simulink model "kopter_se_zavazim_state_feedback"  (R2024b)
settings: Solver=FixedStepAuto  StartTime=0.0  StopTime=30  FixedStep=0.01  RelTol=1e-3
values from neighbouring files (symbols this model uses):
  b_moment = 5.4e-6    (= 5.4e-06)    [parametry_kopter_se_zavazim.m]
  d = 1    [parametry_kopter_se_zavazim.m]
  g = 9.81    [parametry_kopter_se_zavazim.m]
  Ip = m*d^2    (= 1)    [parametry_kopter_se_zavazim.m]
  Ixx = 0.0222    [parametry_kopter_se_zavazim.m]
  Iyy = 0.0222    [parametry_kopter_se_zavazim.m]
  Izz = 0.0429    [parametry_kopter_se_zavazim.m]
  k_thrust = 2.3e-3    (= 0.0023)    [parametry_kopter_se_zavazim.m]
  ki = K_ex(:,17:20)    [odvozeni_stavova_regulace.m]
  ki_oa = K_ex_other_angles(:,17:20)    [odvozeni_stavova_regulace_OTHER_ANGLES.m]
  kp = K_ex(:, 1:16)    [odvozeni_stavova_regulace.m]
  kp_oa = K_ex_other_angles(:, 1:16)    [odvozeni_stavova_regulace_OTHER_ANGLES.m]
  M = 2    [parametry_kopter_se_zavazim.m]
  m = 1    [parametry_kopter_se_zavazim.m]
  Us_p = [(M+m)*g; 0; 0; 0]    [parametry_kopter_se_zavazim.m]
  Xinit_ss = [Xinit_matrix; [0 0 0 0 0 0 0 0]']    [parametry_kopter_se_zavazim.m]
  Xs_p = [0;0;0; 0;0;0; 0;0; 0;0;0; 0;0;0; 0;0]    [parametry_kopter_se_zavazim.m]
undefined symbols (not defined in the file or in its folder): L
libraries: simulink_extras x10
(part 1 of 6)
settings Model: Creator=Admin  LastModifiedBy=Admin

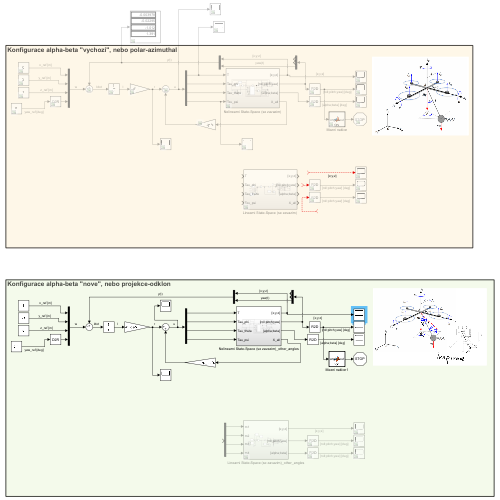
[thumbnail: Simulink's stored preview of the top-level diagram]
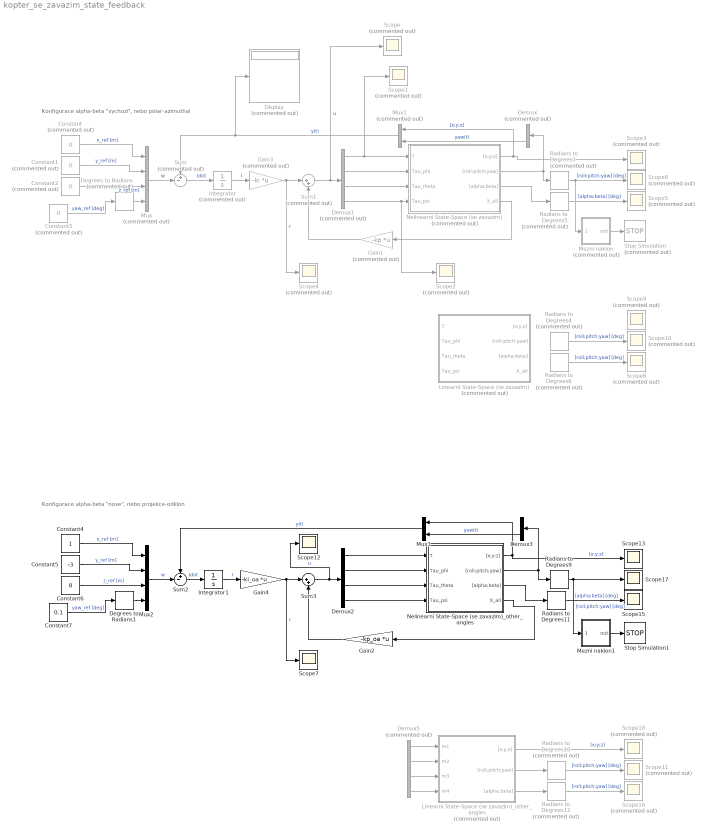
== system kopter_se_zavazim_state_feedback ==
  note: Konfigurace alpha-beta "vychozi", nebo polar-azimuthal
  note: Konfigurace alpha-beta "nove", nebo projekce-odklon
  Constant{,1..3} (4 alike) : Constant  Commented=on  Value=0
  Constant4 : Constant
  Constant5 : Constant  Value=-3
  Constant6 : Constant  Value=8
  Constant7 : Constant  Value=0.1
  Degrees to Radians : simulink_extras/Transformations/Degrees to Radians  Commented=on
  Degrees to Radians1 : simulink_extras/Transformations/Degrees to Radians
  Demux : Demux  Commented=on  Outputs=3
  Demux1 : Demux  Commented=on
  Demux2 : Demux
  Demux3 : Demux  Outputs=3
  Demux5 : Demux  Commented=on
  Display : Display  Commented=on
  Gain1 : Gain  Commented=on  Gain=-kp  Multiplication=Matrix(K*u)
  Gain2 : Gain  Gain=-kp_oa  Multiplication=Matrix(K*u)
  Gain3 : Gain  Commented=on  Gain=-ki  Multiplication=Matrix(K*u)
  Gain4 : Gain  Gain=-ki_oa  Multiplication=Matrix(K*u)
  Integrator : Integrator  Commented=on
  Integrator1 : Integrator
  "Linearni State-Space (se zavazim) " : Subsystem  Commented=on
  Linearni State-Space (se zavazim)_other_angles : Subsystem  Commented=on
  Mezni naklon : MATLAB Function  Commented=on  TreatAsAtomicUnit=on
  Mezni naklon1 : MATLAB Function  TreatAsAtomicUnit=on
  Mux : Mux  Commented=on
  Mux1 : Mux  Commented=on  Inputs=2
  Mux2 : Mux
  Mux3 : Mux  Inputs=2
  Nelinearni State-Space (se zavazim) : Subsystem  Commented=on
  Nelinearni State-Space (se zavazim)_other_angles : Subsystem
  Radians to Degrees{3..6,10,12} (6 alike) : simulink_extras/Transformations/Radians to Degrees  Commented=on
  Radians to Degrees11 : simulink_extras/Transformations/Radians to Degrees
  Radians to Degrees9 : simulink_extras/Transformations/Radians to Degrees
  Scope{,1..6,8..11,16,18} (13 alike) : Scope  Commented=on
  Scope{7,12..13,15,17} (5 alike) : Scope
  Stop Simulation : Stop  Commented=on
  Stop Simulation1 : Stop
  Sum : Sum  Commented=on  Inputs=+-|
  Sum1 : Sum  Commented=on  Inputs=|++
  Sum2 : Sum  Inputs=+-|
  Sum3 : Sum  Inputs=|++
  wires:
  Linearni State-Space (se zavazim)_other_angles/1("[x;y;z]") -> Scope18/1  "[x;y;z]"
  Nelinearni State-Space (se zavazim)/2("[roll;pitch;yaw]") -> Radians to Degrees3/1, Demux/1
  Demux5/3 -> Linearni State-Space (se zavazim)_other_angles/3(m3)
  Radians to Degrees6/1 -> Scope6/1  "[roll;pitch;yaw] [deg]"
  ? -> Radians to Degrees6/1
  Demux5/2 -> Linearni State-Space (se zavazim)_other_angles/2(m2)
  Radians to Degrees5/1 -> Scope5/1  "[alpha;beta] [deg]"
  Nelinearni State-Space (se zavazim)_other_angles/3("[alpha;beta]") -> Radians to Degrees11/1
  ? -> Radians to Degrees4/1
  Linearni State-Space (se zavazim)_other_angles/3("[alpha;beta]") -> Radians to Degrees12/1
  Radians to Degrees10/1 -> Scope11/1  "[roll;pitch;yaw] [deg]"
  Radians to Degrees3/1 -> Mezni naklon/1(angles), Scope8/1  "[roll;pitch;yaw] [deg]"
  Linearni State-Space (se zavazim)_other_angles/2("[roll;pitch;yaw]") -> Radians to Degrees10/1
  Radians to Degrees12/1 -> Scope16/1  "[roll;pitch;yaw] [deg]"
  Demux5/1 -> Linearni State-Space (se zavazim)_other_angles/1(m1)
  Demux5/4 -> Linearni State-Space (se zavazim)_other_angles/4(m4)
  Nelinearni State-Space (se zavazim)/1("[x;y;z]") -> Mux1/1, Scope3/1  "[x;y;z]"
  Radians to Degrees4/1 -> Scope10/1  "[roll;pitch;yaw] [deg]"
  ? -> Scope9/1  "[x;y;z]"
  Radians to Degrees9/1 -> Mezni naklon1/1(angles), Scope17/1  "[roll;pitch;yaw] [deg]"
  Radians to Degrees11/1 -> Scope15/1  "[alpha;beta] [deg]"
  Nelinearni State-Space (se zavazim)/3("[alpha;beta]") -> Radians to Degrees5/1
  Constant/1 -> Mux/1  "x_ref [m]"
  Constant1/1 -> Mux/2  "y_ref [m]"
  Constant2/1 -> Mux/3  "z_ref [m]"
  Degrees to Radians/1 -> Mux/4
  Constant3/1 -> Degrees to Radians/1  "yaw_ref [deg]"
  Mux/1 -> Sum/2  "w"
  Demux/3 -> Mux1/2  "yaw(t)"
  Mux1/1 -> Display/1, Sum/1  "y(t)"
  Sum/1 -> Integrator/1  "Idot"
  Integrator/1 -> Gain3/1  "I"
  Gain3/1 -> Scope4/1, Sum1/1  "r"
  Gain1/1 -> Sum1/2
  Sum1/1 -> Scope/1, Demux1/1  "u"
  Demux1/1 -> Scope1/1, Nelinearni State-Space (se zavazim)/1(T)
  Demux1/2 -> Nelinearni State-Space (se zavazim)/2(Tau_phi)
  Demux1/3 -> Nelinearni State-Space (se zavazim)/3(Tau_theta)
  Demux1/4 -> Nelinearni State-Space (se zavazim)/4(Tau_psi), Scope2/1
  Nelinearni State-Space (se zavazim)/4(X_all) -> Gain1/1
  Mezni naklon/1(out) -> Stop Simulation/1
  Demux2/3 -> Nelinearni State-Space (se zavazim)_other_angles/3(Tau_theta)
  Demux2/2 -> Nelinearni State-Space (se zavazim)_other_angles/2(Tau_phi)
  Constant5/1 -> Mux2/2  "y_ref [m]"
  Constant7/1 -> Degrees to Radians1/1  "yaw_ref [deg]"
  Constant6/1 -> Mux2/3  "z_ref [m]"
  Gain2/1 -> Sum3/2
  Mux2/1 -> Sum2/2  "w"
  Sum3/1 -> Scope12/1, Demux2/1  "u"
  Mux3/1 -> Sum2/1  "y(t)"
  Demux2/4 -> Nelinearni State-Space (se zavazim)_other_angles/4(Tau_psi)
  Sum2/1 -> Integrator1/1  "Idot"
  Gain4/1 -> Scope7/1, Sum3/1  "r"
  Demux2/1 -> Nelinearni State-Space (se zavazim)_other_angles/1(T)
  Integrator1/1 -> Gain4/1  "I"
  Degrees to Radians1/1 -> Mux2/4
  Constant4/1 -> Mux2/1  "x_ref [m]"
  Demux3/3 -> Mux3/2  "yaw(t)"
  Nelinearni State-Space (se zavazim)_other_angles/1("[x;y;z]") -> Scope13/1, Mux3/1  "[x;y;z]"
  Nelinearni State-Space (se zavazim)_other_angles/2("[roll;pitch;yaw]") -> Radians to Degrees9/1, Demux3/1
  Nelinearni State-Space (se zavazim)_other_angles/4(X_all) -> Gain2/1
  Mezni naklon1/1(out) -> Stop Simulation1/1

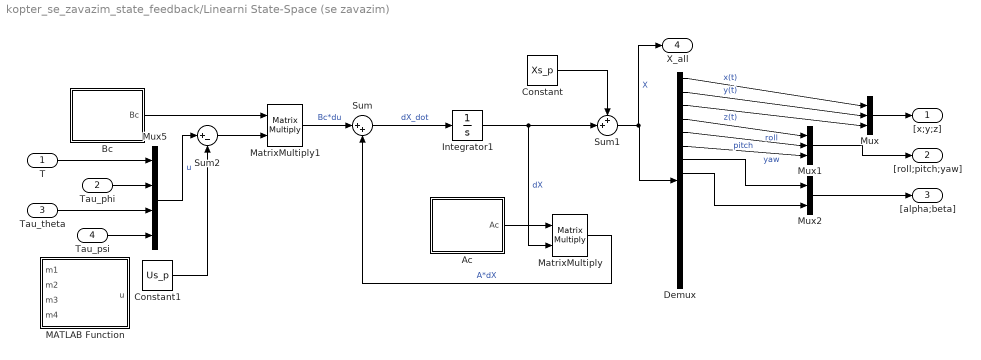
== system kopter_se_zavazim_state_feedback/Linearni State-Space (se zavazim)  ==
  T : Inport
  Tau_phi : Inport  Port=2
  Tau_theta : Inport  Port=3
  Tau_psi : Inport  Port=4
  Ac : MATLAB Function  TreatAsAtomicUnit=on
  Bc : MATLAB Function  TreatAsAtomicUnit=on
  Constant : Constant  Value=Xs_p
  Constant1 : Constant  Value=Us_p
  Demux : Demux  Outputs=16
  Integrator1 : Integrator  InitialCondition=Xinit_ss
  MATLAB Function : MATLAB Function  TreatAsAtomicUnit=on
  MatrixMultiply : Product  Multiplication=Matrix(*)
  MatrixMultiply1 : Product  Multiplication=Matrix(*)
  Mux : Mux  Inputs=3
  Mux1 : Mux  Inputs=3
  Mux2 : Mux  Inputs=2
  Mux5 : Mux
  Sum : Sum  Inputs=|++
  Sum1 : Sum  Inputs=++|
  Sum2 : Sum  Inputs=|+-
  "[x;y;z]" : Outport
  "[roll;pitch;yaw]" : Outport  Port=2
  "[alpha;beta]" : Outport  Port=3
  X_all : Outport  Port=4
  wires:
  Ac/1(Ac) -> MatrixMultiply/1
  Integrator1/1 -> Sum1/2, MatrixMultiply/2  "dX"
  Demux/1 -> Mux/1  "x(t)"
  Demux/2 -> Mux/2  "y(t)"
  Demux/3 -> Mux/3  "z(t)"
  Mux/1 -> "[x;y;z]"/1
  Demux/4 -> Mux1/1  "roll"
  Demux/5 -> Mux1/2  "pitch"
  Demux/6 -> Mux1/3  "yaw"
  Mux1/1 -> "[roll;pitch;yaw]"/1
  Sum/1 -> Integrator1/1  "dX_dot"
  MatrixMultiply1/1 -> Sum/1  "Bc*du"
  MatrixMultiply/1 -> Sum/2  "A*dX"
  Bc/1(Bc) -> MatrixMultiply1/1
  Sum1/1 -> X_all/1, Demux/1  "X"
  Constant/1 -> Sum1/1
  Constant1/1 -> Sum2/2
  Sum2/1 -> MatrixMultiply1/2
  Mux2/1 -> "[alpha;beta]"/1
  Demux/7 -> Mux2/1
  Demux/8 -> Mux2/2
  Tau_theta/1 -> Mux5/3
  Tau_psi/1 -> Mux5/4
  Tau_phi/1 -> Mux5/2
  Mux5/1 -> Sum2/1  "u"
  T/1 -> Mux5/1

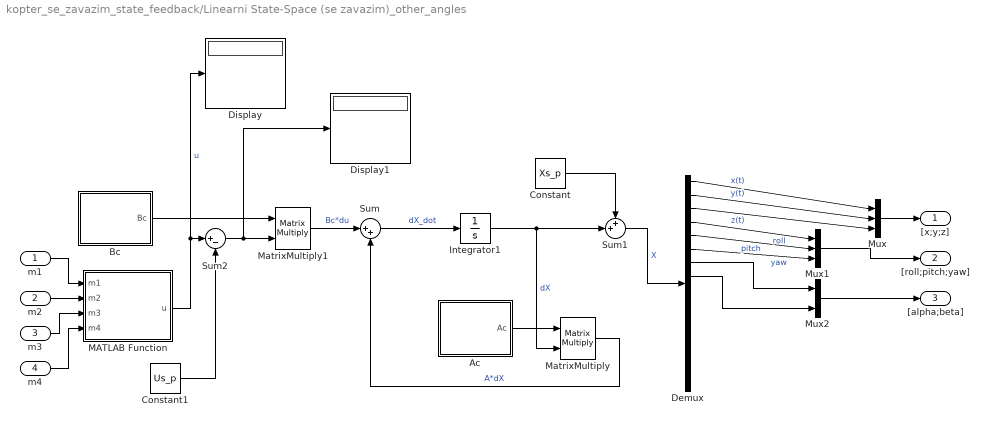
== system kopter_se_zavazim_state_feedback/Linearni State-Space (se zavazim)_other_angles ==
  m1 : Inport
  m2 : Inport  Port=2
  m3 : Inport  Port=3
  m4 : Inport  Port=4
  Ac : MATLAB Function  TreatAsAtomicUnit=on
  Bc : MATLAB Function  TreatAsAtomicUnit=on
  Constant : Constant  Value=Xs_p
  Constant1 : Constant  Value=Us_p
  Demux : Demux  Outputs=16
  Display : Display
  Display1 : Display
  Integrator1 : Integrator  InitialCondition=Xinit_ss
  MATLAB Function : MATLAB Function  TreatAsAtomicUnit=on
  MatrixMultiply : Product  Multiplication=Matrix(*)
  MatrixMultiply1 : Product  Multiplication=Matrix(*)
  Mux : Mux  Inputs=3
  Mux1 : Mux  Inputs=3
  Mux2 : Mux  Inputs=2
  Sum : Sum  Inputs=|++
  Sum1 : Sum  Inputs=++|
  Sum2 : Sum  Inputs=|+-
  "[x;y;z]" : Outport
  "[roll;pitch;yaw]" : Outport  Port=2
  "[alpha;beta]" : Outport  Port=3
  wires:
  MATLAB Function/1(u) -> Display/1, Sum2/1  "u"
  m3/1 -> MATLAB Function/3(m3)
  m2/1 -> MATLAB Function/2(m2)
  m4/1 -> MATLAB Function/4(m4)
  m1/1 -> MATLAB Function/1(m1)
  Ac/1(Ac) -> MatrixMultiply/1
  Integrator1/1 -> Sum1/2, MatrixMultiply/2  "dX"
  Demux/1 -> Mux/1  "x(t)"
  Demux/2 -> Mux/2  "y(t)"
  Demux/3 -> Mux/3  "z(t)"
  Mux/1 -> "[x;y;z]"/1
  Demux/4 -> Mux1/1  "roll"
  Demux/5 -> Mux1/2  "pitch"
  Demux/6 -> Mux1/3  "yaw"
  Mux1/1 -> "[roll;pitch;yaw]"/1
  Sum/1 -> Integrator1/1  "dX_dot"
  MatrixMultiply1/1 -> Sum/1  "Bc*du"
  MatrixMultiply/1 -> Sum/2  "A*dX"
  Bc/1(Bc) -> MatrixMultiply1/1
  Sum1/1 -> Demux/1  "X"
  Constant/1 -> Sum1/1
  Constant1/1 -> Sum2/2
  Sum2/1 -> Display1/1, MatrixMultiply1/2
  Mux2/1 -> "[alpha;beta]"/1
  Demux/7 -> Mux2/1
  Demux/8 -> Mux2/2

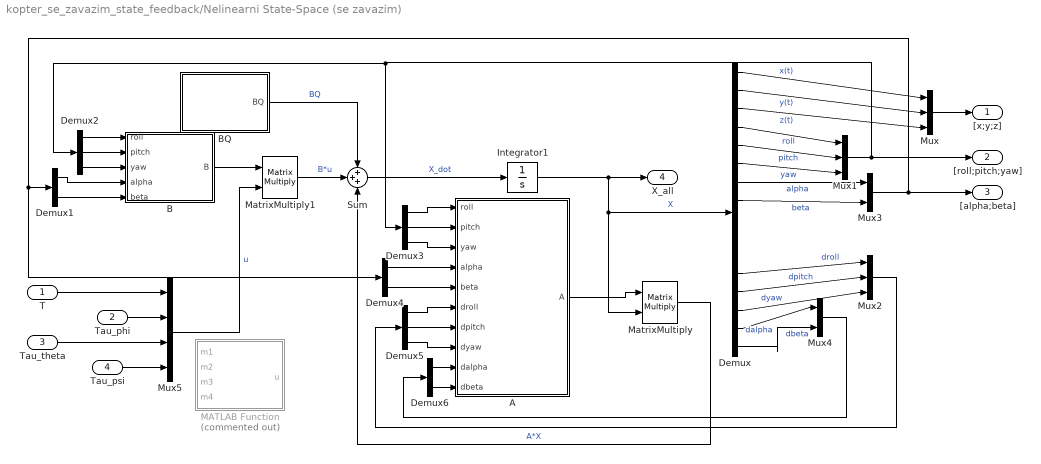
== system kopter_se_zavazim_state_feedback/Nelinearni State-Space (se zavazim) ==
  T : Inport
  Tau_phi : Inport  Port=2
  Tau_theta : Inport  Port=3
  Tau_psi : Inport  Port=4
  A : MATLAB Function  TreatAsAtomicUnit=on
  B : MATLAB Function  TreatAsAtomicUnit=on
  BQ : MATLAB Function  TreatAsAtomicUnit=on
  Demux : Demux  Outputs=16
  Demux1 : Demux  Outputs=2
  Demux2 : Demux  Outputs=3
  Demux3 : Demux  Outputs=3
  Demux4 : Demux  Outputs=2
  Demux5 : Demux  Outputs=3
  Demux6 : Demux  Outputs=2
  Integrator1 : Integrator  InitialCondition=Xinit_ss
  MATLAB Function : MATLAB Function  Commented=on  TreatAsAtomicUnit=on
  MatrixMultiply : Product  Multiplication=Matrix(*)
  MatrixMultiply1 : Product  Multiplication=Matrix(*)
  Mux : Mux  Inputs=3
  Mux1 : Mux  Inputs=3
  Mux2 : Mux  Inputs=3
  Mux3 : Mux  Inputs=2
  Mux4 : Mux  Inputs=2
  Mux5 : Mux
  Sum : Sum  Inputs=+++
  "[x;y;z]" : Outport
  "[roll;pitch;yaw]" : Outport  Port=2
  "[alpha;beta]" : Outport  Port=3
  X_all : Outport  Port=4
  wires:
  Mux5/1 -> MatrixMultiply1/2  "u"
  A/1(A) -> MatrixMultiply/1
  Integrator1/1 -> X_all/1, MatrixMultiply/2, Demux/1  "X"
  Demux/1 -> Mux/1  "x(t)"
  Demux/2 -> Mux/2  "y(t)"
  Demux/3 -> Mux/3  "z(t)"
  Mux/1 -> "[x;y;z]"/1
  Demux/4 -> Mux1/1  "roll"
  Demux/5 -> Mux1/2  "pitch"
  Demux/6 -> Mux1/3  "yaw"
  Mux1/1 -> Demux2/1, Demux3/1, "[roll;pitch;yaw]"/1
  Demux/12 -> Mux2/1  "droll"
  Demux/13 -> Mux2/2  "dpitch"
  Demux/14 -> Mux2/3  "dyaw"
  Demux2/1 -> B/1(roll)
  Demux2/2 -> B/2(pitch)
  Demux2/3 -> B/3(yaw)
  Demux3/2 -> A/2(pitch)
  Demux3/1 -> A/1(roll)
  Demux3/3 -> A/3(yaw)
  Demux5/2 -> A/7(dpitch)
  Demux5/1 -> A/6(droll)
  Demux5/3 -> A/8(dyaw)
  Sum/1 -> Integrator1/1  "X_dot"
  BQ/1(BQ) -> Sum/1  "BQ"
  MatrixMultiply1/1 -> Sum/2  "B*u"
  B/1(B) -> MatrixMultiply1/1
  MatrixMultiply/1 -> Sum/3  "A*X"
  Mux2/1 -> Demux5/1
  Demux/7 -> Mux3/1  "alpha"
  Demux/8 -> Mux3/2  "beta"
  Mux3/1 -> Demux4/1, Demux1/1, "[alpha;beta]"/1
  Demux1/2 -> B/5(beta)
  Demux1/1 -> B/4(alpha)
  Demux4/2 -> A/5(beta)
  Demux4/1 -> A/4(alpha)
  Demux/15 -> Mux4/1  "dalpha"
  Demux/16 -> Mux4/2  "dbeta"
  Demux6/1 -> A/9(dalpha)
  Demux6/2 -> A/10(dbeta)
  Mux4/1 -> Demux6/1
  T/1 -> Mux5/1
  Tau_phi/1 -> Mux5/2
  Tau_theta/1 -> Mux5/3
  Tau_psi/1 -> Mux5/4

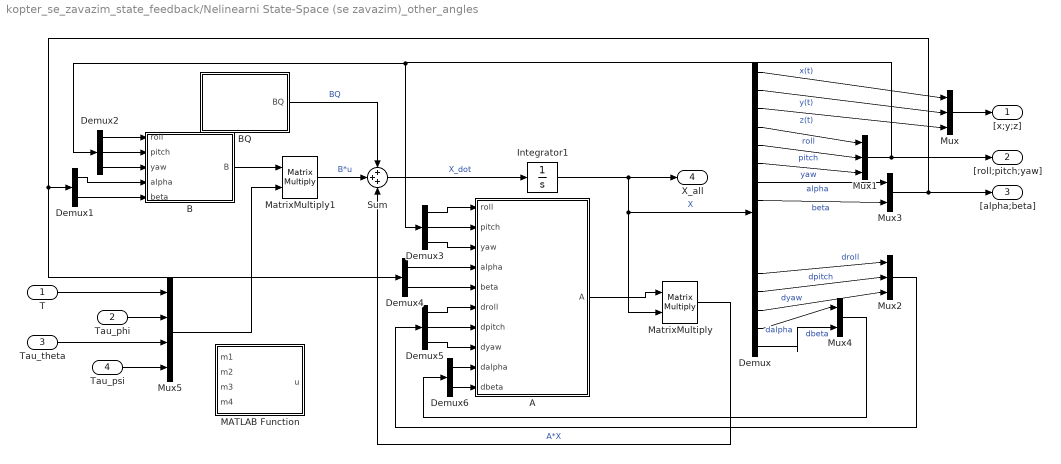
== system kopter_se_zavazim_state_feedback/Nelinearni State-Space (se zavazim)_other_angles ==
  T : Inport
  Tau_phi : Inport  Port=2
  Tau_theta : Inport  Port=3
  Tau_psi : Inport  Port=4
  A : MATLAB Function  TreatAsAtomicUnit=on
  B : MATLAB Function  TreatAsAtomicUnit=on
  BQ : MATLAB Function  TreatAsAtomicUnit=on
  Demux : Demux  Outputs=16
  Demux1 : Demux  Outputs=2
  Demux2 : Demux  Outputs=3
  Demux3 : Demux  Outputs=3
  Demux4 : Demux  Outputs=2
  Demux5 : Demux  Outputs=3
  Demux6 : Demux  Outputs=2
  Integrator1 : Integrator  InitialCondition=Xinit_ss
  MATLAB Function : MATLAB Function  TreatAsAtomicUnit=on
  MatrixMultiply : Product  Multiplication=Matrix(*)
  MatrixMultiply1 : Product  Multiplication=Matrix(*)
  Mux : Mux  Inputs=3
  Mux1 : Mux  Inputs=3
  Mux2 : Mux  Inputs=3
  Mux3 : Mux  Inputs=2
  Mux4 : Mux  Inputs=2
  Mux5 : Mux
  Sum : Sum  Inputs=+++
  "[x;y;z]" : Outport
  "[roll;pitch;yaw]" : Outport  Port=2
  "[alpha;beta]" : Outport  Port=3
  X_all : Outport  Port=4
  wires:
  A/1(A) -> MatrixMultiply/1
  Integrator1/1 -> MatrixMultiply/2, Demux/1, X_all/1  "X"
  Demux/1 -> Mux/1  "x(t)"
  Demux/2 -> Mux/2  "y(t)"
  Demux/3 -> Mux/3  "z(t)"
  Mux/1 -> "[x;y;z]"/1
  Demux/4 -> Mux1/1  "roll"
  Demux/5 -> Mux1/2  "pitch"
  Demux/6 -> Mux1/3  "yaw"
  Mux1/1 -> Demux2/1, Demux3/1, "[roll;pitch;yaw]"/1
  Demux/12 -> Mux2/1  "droll"
  Demux/13 -> Mux2/2  "dpitch"
  Demux/14 -> Mux2/3  "dyaw"
  Demux2/1 -> B/1(roll)
  Demux2/2 -> B/2(pitch)
  Demux2/3 -> B/3(yaw)
  Demux3/2 -> A/2(pitch)
  Demux3/1 -> A/1(roll)
  Demux3/3 -> A/3(yaw)
  Demux5/2 -> A/7(dpitch)
  Demux5/1 -> A/6(droll)
  Demux5/3 -> A/8(dyaw)
  Sum/1 -> Integrator1/1  "X_dot"
  BQ/1(BQ) -> Sum/1  "BQ"
  MatrixMultiply1/1 -> Sum/2  "B*u"
  B/1(B) -> MatrixMultiply1/1
  MatrixMultiply/1 -> Sum/3  "A*X"
  Mux2/1 -> Demux5/1
  Demux/7 -> Mux3/1  "alpha"
  Demux/8 -> Mux3/2  "beta"
  Mux3/1 -> Demux4/1, Demux1/1, "[alpha;beta]"/1
  Demux1/2 -> B/5(beta)
  Demux1/1 -> B/4(alpha)
  Demux4/2 -> A/5(beta)
  Demux4/1 -> A/4(alpha)
  Demux/15 -> Mux4/1  "dalpha"
  Demux/16 -> Mux4/2  "dbeta"
  Demux6/1 -> A/9(dalpha)
  Demux6/2 -> A/10(dbeta)
  Mux4/1 -> Demux6/1
  Tau_theta/1 -> Mux5/3
  Tau_psi/1 -> Mux5/4
  Tau_phi/1 -> Mux5/2
  Mux5/1 -> MatrixMultiply1/2
  T/1 -> Mux5/1

== matlab function kopter_se_zavazim_state_feedback/Nelinearni State-Space (se zavazim)/MATLAB Function ==
  data: u output; m1 input; m2 input; m3 input; m4 input; k_thrust parameter; b_moment parameter; L parameter
function u = fcn(m1, m2, m3, m4, k_thrust, b_moment, L)

Thrust = k_thrust*(m1^2 + m2^2 + m3^2 + m4^2);
Tau_roll = L*k_thrust*(m1^2 + m4^2 - m2^2 - m3^2);
Tau_pitch = L*k_thrust*(m4^2 + m3^2 - m1^2 - m2^2);
Tau_yaw = b_moment*(m1^2 + m3^2 - m2^2 - m4^2);

u = [Thrust; Tau_roll; Tau_pitch; Tau_yaw];

== matlab function kopter_se_zavazim_state_feedback/Linearni State-Space (se zavazim) /Bc ==
  data: M parameter; Bc output; Ixx parameter; Iyy parameter; Izz parameter; m parameter
function Bc = fcn(M, Ixx, Iyy, Izz, m)
% Matice Ac linearizovana

Bc = [
        0,     0,     0,     0;
        0,     0,     0,     0;
        0,     0,     0,     0;
        0,     0,     0,     0;
        0,     0,     0,     0;
        0,     0,     0,     0;
        0,     0,     0,     0;
        0,     0,     0,     0;
        0,     0,     0,     0;
        0,     0,     0,     0;
1/(M + m),     0,     0,     0;
        0, 1/Ixx,     0,     0;
        0,     0, 1/Iyy,     0;
        0,     0,     0, 1/Izz;
        0,     0,     0,     0;
        0,     0,     0,     0];
